simulink model "ats"  (Simulink 8.8)
settings: Solver=FixedStepDiscrete  StartTime=0.0  StopTime=10.0  FixedStep=0.1  RelTol=1e-3  EnableMultiTasking=on
settings Model: Creator=think  LastModifiedBy=think
settings SolverCC: AutoInsertRateTranBlk=on
settings DataIOCC: SaveFormat=Dataset  SignalLoggingSaveFormat=Dataset
settings DebuggingCC: UnderspecifiedInitializationDetection=Simplified  MergeDetectMultiDrivingBlocksExec=error  FcnCallInpInsideContextMsg=error  AllowSymbolicDim=off  StateNameClashWarn=none
settings HardwareCC: ProdBitPerPointer=64  ProdBitPerSizeT=64  ProdBitPerPtrDiffT=64  ProdLargestAtomicFloat=Float  ProdIntDivRoundTo=Zero  ProdEndianess=LittleEndian  ProdWordSize=64  ProdHWDeviceType=Intel->x86-64 (Windows64)
settings ModelReferenceCC: PropagateSignalLabelsOutOfModel=on
settings GRTTargetCC: CombineOutputUpdateFcns=on  GRTInterface=off
settings ConfigComp: CovSFcnEnable=off

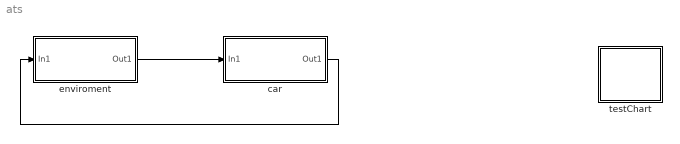
== system ats ==
  car : Subsystem
  enviroment : Subsystem
  testChart : Stateflow chart  TreatAsAtomicUnit=on
  wires:
  enviroment/1(Out1) -> car/1(In1)
  car/1(Out1) -> enviroment/1(In1)

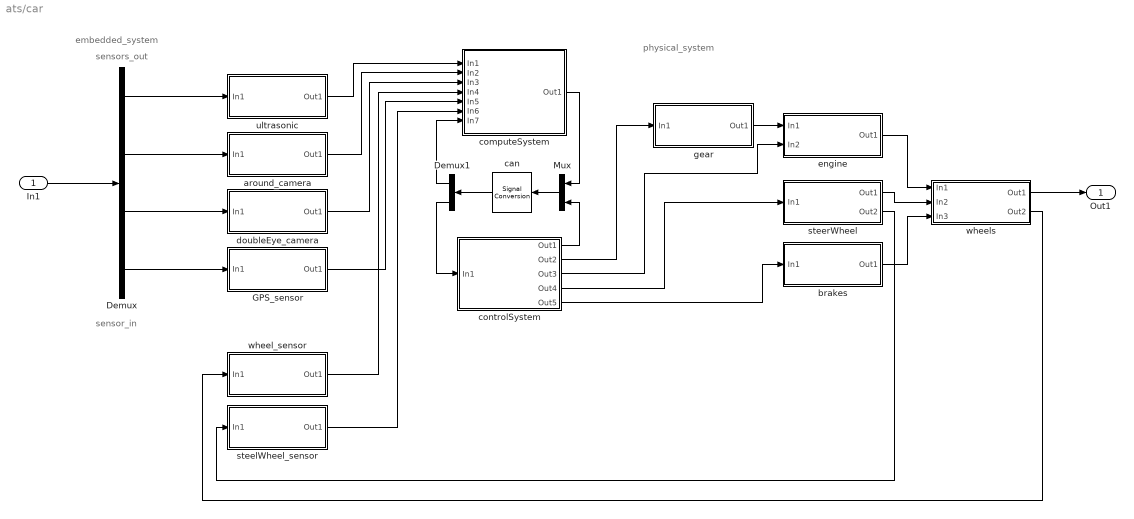
== system ats/car ==
  note: sensor_in
  note: physical_system
  note: embedded_system
  note: sensors_out
  In1 : Inport
  Demux : Demux
  Demux1 : Demux  Outputs=2
  GPS_sensor : Subsystem
  Mux : Mux  Inputs=2
  around_camera : Subsystem
  brakes : Subsystem
  can : SignalConversion  ConversionOutput=Nonvirtual bus  OutDataTypeStr=Bus: can  OverrideOpt=off
  computeSystem : Subsystem
  controlSystem : Subsystem
  doubleEye_camera : Subsystem
  engine : Subsystem
  gear : Subsystem
  steelWheel_sensor : Subsystem
  steerWheel : Subsystem
  ultrasonic : Subsystem
  wheel_sensor : Subsystem
  "wheels " : Subsystem
  Out1 : Outport
  wires:
  In1/1 -> Demux/1
  Demux/1 -> ultrasonic/1(In1)
  Demux/3 -> doubleEye_camera/1(In1)
  Demux/2 -> around_camera/1(In1)
  Mux/1 -> can/1
  can/1 -> Demux1/1
  computeSystem/1(Out1) -> Mux/1
  controlSystem/1(Out1) -> Mux/2
  Demux1/1 -> computeSystem/7(In7)
  Demux1/2 -> controlSystem/1(In1)
  gear/1(Out1) -> engine/1(In1)
  steerWheel/1(Out1) -> "wheels "/2(In2)
  engine/1(Out1) -> "wheels "/1(In1)
  brakes/1(Out1) -> "wheels "/3(In3)
  controlSystem/2(Out2) -> gear/1(In1)
  controlSystem/4(Out4) -> steerWheel/1(In1)
  controlSystem/3(Out3) -> engine/2(In2)
  "wheels "/1(Out1) -> Out1/1
  ultrasonic/1(Out1) -> computeSystem/1(In1)
  around_camera/1(Out1) -> computeSystem/2(In2)
  doubleEye_camera/1(Out1) -> computeSystem/3(In3)
  wheel_sensor/1(Out1) -> computeSystem/4(In4)
  GPS_sensor/1(Out1) -> computeSystem/5(In5)
  steelWheel_sensor/1(Out1) -> computeSystem/6(In6)
  steerWheel/2(Out2) -> steelWheel_sensor/1(In1)
  "wheels "/2(Out2) -> wheel_sensor/1(In1)
  Demux/4 -> GPS_sensor/1(In1)
  controlSystem/5(Out5) -> brakes/1(In1)

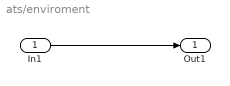
== system ats/enviroment ==
  In1 : Inport
  Out1 : Outport
  wires:
  In1/1 -> Out1/1

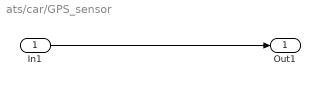
== system ats/car/GPS_sensor ==
  In1 : Inport
  Out1 : Outport
  wires:
  In1/1 -> Out1/1

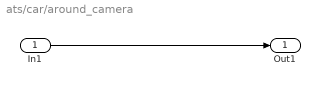
== system ats/car/around_camera ==
  In1 : Inport
  Out1 : Outport
  wires:
  In1/1 -> Out1/1

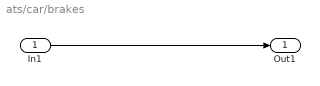
== system ats/car/brakes ==
  In1 : Inport
  Out1 : Outport
  wires:
  In1/1 -> Out1/1

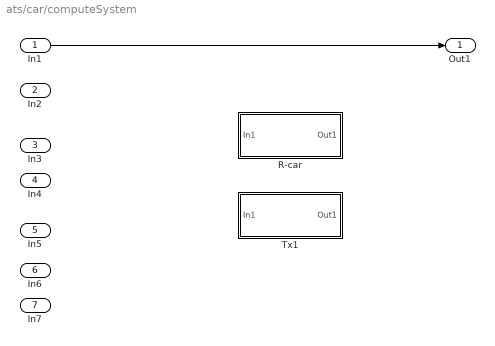
== system ats/car/computeSystem ==
  In1 : Inport
  In2 : Inport  Port=2
  In3 : Inport  Port=3
  In4 : Inport  Port=4
  In5 : Inport  Port=5
  In6 : Inport  Port=6
  In7 : Inport  Port=7
  R-car : Subsystem
  Tx1 : Subsystem
  Out1 : Outport
  wires:
  In1/1 -> Out1/1

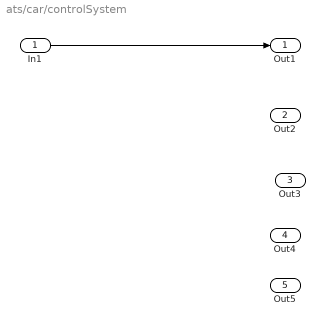
== system ats/car/controlSystem ==
  In1 : Inport
  Out1 : Outport
  Out2 : Outport  Port=2
  Out3 : Outport  Port=3
  Out4 : Outport  Port=4
  Out5 : Outport  Port=5
  wires:
  In1/1 -> Out1/1

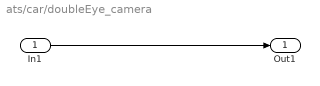
== system ats/car/doubleEye_camera ==
  In1 : Inport
  Out1 : Outport
  wires:
  In1/1 -> Out1/1

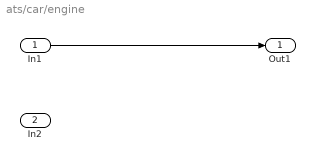
== system ats/car/engine ==
  In1 : Inport
  In2 : Inport  Port=2
  Out1 : Outport
  wires:
  In1/1 -> Out1/1

== system ats/car/gear ==
  In1 : Inport
  Out1 : Outport
  wires:
  In1/1 -> Out1/1

== system ats/car/steelWheel_sensor ==
  In1 : Inport
  Out1 : Outport
  wires:
  In1/1 -> Out1/1

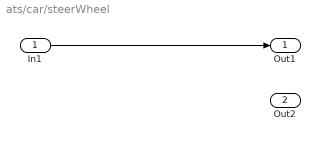
== system ats/car/steerWheel ==
  In1 : Inport
  Out1 : Outport
  Out2 : Outport  Port=2
  wires:
  In1/1 -> Out1/1

== system ats/car/ultrasonic ==
  In1 : Inport
  Out1 : Outport
  wires:
  In1/1 -> Out1/1

== system ats/car/wheel_sensor ==
  In1 : Inport
  Out1 : Outport
  wires:
  In1/1 -> Out1/1

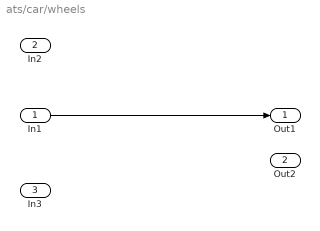
== system ats/car/wheels  ==
  In1 : Inport
  In2 : Inport  Port=2
  In3 : Inport  Port=3
  Out1 : Outport
  Out2 : Outport  Port=2
  wires:
  In1/1 -> Out1/1

== system ats/car/computeSystem/R-car ==
  In1 : Inport
  Out1 : Outport
  wires:
  In1/1 -> Out1/1

== system ats/car/computeSystem/Tx1 ==
  In1 : Inport
  Out1 : Outport
  wires:
  In1/1 -> Out1/1

== stateflow chart testChart ==
  state ComputeSystem [group]
    state R_car
    state Tx1
  state sensors [group]
    state ultrasonic
    state aroundCamera
    state eyeCamera
  state EnviromentMoniter [group]
    state barreir
    state stopPlace
    state stopSign
    (default) -> barreir
  state Actuators [group]
  state ControlSystem [group]
  barreir -> ultrasonic
  ultrasonic -> R_car
  aroundCamera -> R_car
  stopPlace -> aroundCamera
  eyeCamera -> Tx1
  stopSign -> eyeCamera
